simulink model "Model_v2"  (R2021a)
settings: Solver=ode23tb  StartTime=0.0  StopTime=10  FixedStep=1e-3  RelTol=1e-3
undefined symbols (not defined in the file): j1, j2d, j2u, j3d, j3u, j4, j5, Levenberg, Marquardt, X, Y, Z
libraries: sm_lib x37, nesl_utility x13, simulink_extras x12, pid_lib x6, robotmaniplib x1, robotcorelib x1
(part 2 of 2)

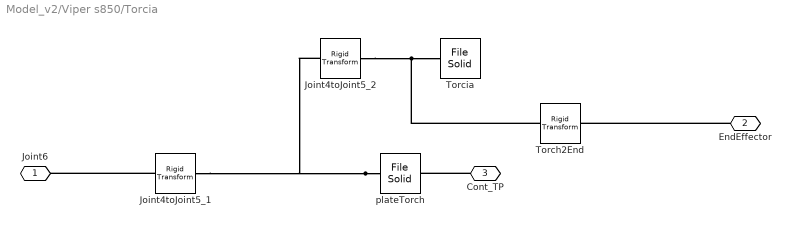
== system Model_v2/Viper s850/Torcia ==
  Joint4toJoint5_1 : sm_lib/Frames and Transforms/Rigid Transform  TranslationMethod=StandardAxis  TranslationStandardOffset=endPlate  TranslationLengthUnit=mm  TranslationStandardAxis=+Z  TranslationCartesianOffset=l5  TranslationROffset=0  TranslationROffsetUnits=m  TranslationZOffset=0  TranslationZOffsetUnits=m  TranslationThetaOffset=0  TranslationThetaOffsetUnits=deg  RotationMethod=None  RotationAngleUnits=deg  RotationStandardAxis=+X  RotationAngle=90  RotationArbitraryAxis=[0 0 1]  FollAlignAxisA=+X  BaseAlignAxisA=+Y  FollAlignAxisB=+Y  BaseAlignAxisB=+Z  RotationSequenceAxes=FollowerAxes  RotationSequence=XYX  RotationSequenceAngles=[0 0 0]  RotationSequenceAnglesUnits=deg  RotationMatrix=[1 0 0; 0 1 0; 0 0 1]
  Joint4toJoint5_2 : sm_lib/Frames and Transforms/Rigid Transform  TranslationMethod=Cartesian  TranslationStandardOffset=endTor  TranslationLengthUnit=mm  TranslationStandardAxis=+Z  TranslationCartesianOffset=endTor  TranslationROffset=0  TranslationROffsetUnits=m  TranslationZOffset=0  TranslationZOffsetUnits=m  TranslationThetaOffset=0  TranslationThetaOffsetUnits=deg  RotationMethod=None  RotationAngleUnits=deg  RotationStandardAxis=+X  RotationAngle=90  RotationArbitraryAxis=[0 0 1]  FollAlignAxisA=+X  BaseAlignAxisA=+Y  FollAlignAxisB=+Y  BaseAlignAxisB=+Z  RotationSequenceAxes=FollowerAxes  RotationSequence=XYX  RotationSequenceAngles=[0 0 0]  RotationSequenceAnglesUnits=deg  RotationMatrix=[1 0 0; 0 1 0; 0 0 1]
  Torch2End : sm_lib/Frames and Transforms/Rigid Transform  TranslationMethod=Cartesian  TranslationStandardOffset=endTor  TranslationLengthUnit=mm  TranslationStandardAxis=+Z  TranslationCartesianOffset=[80 0 420]  TranslationROffset=0  TranslationROffsetUnits=m  TranslationZOffset=0  TranslationZOffsetUnits=m  TranslationThetaOffset=0  TranslationThetaOffsetUnits=deg  RotationMethod=None  RotationAngleUnits=deg  RotationStandardAxis=+X  RotationAngle=90  RotationArbitraryAxis=[0 0 1]  FollAlignAxisA=+X  BaseAlignAxisA=+Y  FollAlignAxisB=+Y  BaseAlignAxisB=+Z  RotationSequenceAxes=FollowerAxes  RotationSequence=XYX  RotationSequenceAngles=[0 0 0]  RotationSequenceAnglesUnits=deg  RotationMatrix=[1 0 0; 0 1 0; 0 0 1]
  Torcia : sm_lib/Body Elements/File Solid  ExtGeomFileName=/home/giulio/Scrivania/PhD/Didattica/ISAPI/1. ESE_SIMULATION/RobotViperS850/WeldingTorch.SLDPRT  UnitType=FromFile  ExtGeomFileUnits=m  StepReaderType=HEX  ExportConvexHullGeometry=off  InertiaType=CalculateFromGeometry  Mass=1  MassUnits=kg  CenterOfMass=[0 0 0]  CenterOfMassUnits=m  MomentsOfInertia=[1 1 1]  MomentsOfInertiaUnits=kg*m^2  ProductsOfInertia=[0 0 0]  ProductsOfInertiaUnits=kg*m^2  BasedOnType=DensityFromFile  Density=1000  DensityUnits=kg/m^3  DoExposeReferenceFrame=on  SerializedFrames=<Frames/>  GraphicType=FromGeometry  MarkerShape=Sphere  MarkerSize=10  GraphicVisPropType=SimpleVisualProperties  GraphicDiffuseColor=[0.6 0.6 0.6]  GraphicSpecularColor=[0.5 0.5 0.5 1.0]  GraphicAmbientColor=[0.15 0.15 0.15 1.0]  GraphicEmissiveColor=[0.0 0.0 0.0 1.0]  GraphicShininess=75  GraphicOpacity=1.0
  plateTorch : sm_lib/Body Elements/File Solid  ExtGeomFileName=/home/giulio/Scrivania/PhD/Didattica/ISAPI/1. ESE_SIMULATION/RobotViperS850/LTorcia.sldprt  UnitType=FromFile  ExtGeomFileUnits=m  StepReaderType=HEX  ExportConvexHullGeometry=on  InertiaType=CalculateFromGeometry  Mass=1  MassUnits=kg  CenterOfMass=[0 0 0]  CenterOfMassUnits=m  MomentsOfInertia=[1 1 1]  MomentsOfInertiaUnits=kg*m^2  ProductsOfInertia=[0 0 0]  ProductsOfInertiaUnits=kg*m^2  BasedOnType=DensityFromFile  Density=1000  DensityUnits=kg/m^3  DoExposeReferenceFrame=on  SerializedFrames=<Frames/>  GraphicType=FromGeometry  MarkerShape=Sphere  MarkerSize=10  GraphicVisPropType=SimpleVisualProperties  GraphicDiffuseColor=[0.6 0.0 0.2]  GraphicSpecularColor=[0.5 0.5 0.5 1.0]  GraphicAmbientColor=[0.15 0.15 0.15 1.0]  GraphicEmissiveColor=[0.0 0.0 0.0 1.0]  GraphicShininess=75  GraphicOpacity=1.0
  Joint6 : PMIOPort  Side=Left
  EndEffector : PMIOPort  Port=2  Side=Right
  Cont_TP : PMIOPort  Port=3  Side=Right
  connections:
  Joint4toJoint5_1/LConn1 -- Joint6/RConn1
  Joint4toJoint5_2/RConn1 -- Torch2End/LConn1 -- Torcia/RConn1
  EndEffector/RConn1 -- Torch2End/RConn1
  Cont_TP/RConn1 -- plateTorch/LConn1
  plateTorch/RConn1 -- Joint4toJoint5_1/RConn1 -- Joint4toJoint5_2/LConn1

== matlab function Model_v2/Controller/Path planning ==
  data: q input; pose output; weights output
function [pose,weights] = pathplanning(q)

pose=[-1,0,0,q(1); 
    0,-1,0, q(2);
    0,0,-1,q(3);
    0,0,0,1];

weights = [1, 1, 1, 1, 1, 1];
